simulink model "rfkjr"  (R2024a)
settings: Solver=FixedStepAuto  StartTime=0.0  StopTime=inf  FixedStep=0.1  RelTol=1e-3
libraries: robotlib x6
settings Model: Creator=ronnie.yalung  LastModifiedBy=ronnie.yalung
settings OptimizationCC: EnhancedBackFolding=on  PassReuseOutputArgsAs=Individual arguments  ZeroExternalMemoryAtStartup=off  ZeroInternalMemoryAtStartup=off  MaxStackSize=64  OptimizeBlockOrder=speed  DifferentSizesBufferReuse=on  OptimizationCustomize=off  EfficientTunableParamExpr=on
settings DebuggingCC: ParameterTunabilityLossMsg=error
settings HardwareCC: ProdBitPerLong=64  ProdHWDeviceType=Apple->ARM64  UseEmbeddedCoderFeatures=off
settings SFSimCC: MATLABDynamicMemAlloc=off
settings RTWCC: Description=Embedded Coder  SystemTargetFile=ert.tlc  HardwareBoard=Robot Operating System 2 (ROS 2)  TLCOptions="-aInlineSetEventsForThisBaseRateFcn=TLC_FALSE -aSuppressMultiTaskScheduler=TLC_FALSE  -aRateBasedStepFcn=0"  TemplateMakefile=ert_default_tmf  Toolchain=Colcon Tools  TargetLang=C++
settings CodeAppCC: ForceParamTrailComments=on  IgnoreCustomStorageClasses=off  OperatorAnnotations=on  SimulinkDataObjDesc=on  SFDataObjDesc=on  InsertBlockDesc=on
settings ERTTargetCC: CodeInterfacePackaging=C++ class  SupportNonInlinedSFcns=on

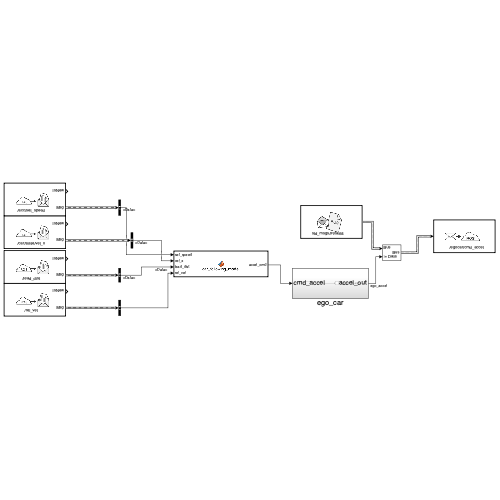
[thumbnail: Simulink's stored preview of the top-level diagram]
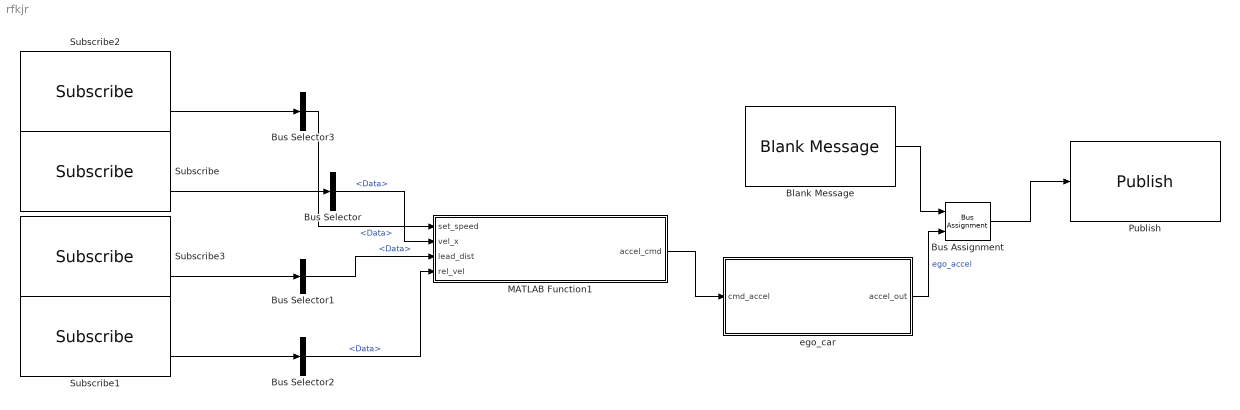
== system rfkjr ==
  Blank Message : robotlib/Blank Message  messageClass=Message  entityType=std_msgs/Float64  messageType=std_msgs/Float64  SampleTime=inf  legacyBusStruct=off
  Bus Assignment : BusAssignment  AssignedSignals=Data
  Bus Selector{,1..3} (4 alike) : BusSelector  OutputSignals=Data
  MATLAB Function1 : MATLAB Function  TreatAsAtomicUnit=on
  Publish : robotlib/Publish  topicSource=Specify your own  topic=/egocar/cmd_accel  messageType=std_msgs/Float64  legacyBusStruct=off  messageQueueLength=1
  Subscribe : robotlib/Subscribe  topicSource=Specify your own  topic=/car/state/vel_x  messageType=std_msgs/Float64  SampleTime=-1  legacyBusStruct=off  messageQueueLength=1
  Subscribe1 : robotlib/Subscribe  topicSource=Specify your own  topic=/rel_vel  messageType=std_msgs/Float64  SampleTime=-1  legacyBusStruct=off  messageQueueLength=1
  Subscribe2 : robotlib/Subscribe  topicSource=Specify your own  topic=/acc/set_speed  messageType=std_msgs/Int16  SampleTime=-1  legacyBusStruct=off  messageQueueLength=1
  Subscribe3 : robotlib/Subscribe  topicSource=Specify your own  topic=/lead_dist  messageType=std_msgs/Float64  SampleTime=-1  legacyBusStruct=off  messageQueueLength=1
  ego_car : Subsystem
  wires:
  MATLAB Function1/1(accel_cmd) -> ego_car/1(cmd_accel)
  Bus Assignment/1 -> Publish/1
  Blank Message/1 -> Bus Assignment/1
  ego_car/1(accel_out) -> Bus Assignment/2  "ego_accel"
  Subscribe/2 -> Bus Selector/1
  Bus Selector/1 -> MATLAB Function1/2(vel_x)  "<Data>"
  Subscribe3/2 -> Bus Selector1/1
  Bus Selector1/1 -> MATLAB Function1/3(lead_dist)  "<Data>"
  Subscribe1/2 -> Bus Selector2/1
  Bus Selector2/1 -> MATLAB Function1/4(rel_vel)  "<Data>"
  Subscribe2/2 -> Bus Selector3/1
  Bus Selector3/1 -> MATLAB Function1/1(set_speed)  "<Data>"

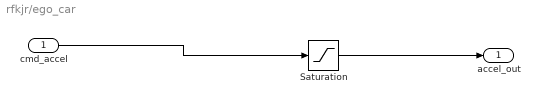
== system rfkjr/ego_car ==
  cmd_accel : Inport
  Saturation : Saturate  UpperLimit=5  LowerLimit=-5
  accel_out : Outport
  wires:
  Saturation/1 -> accel_out/1
  cmd_accel/1 -> Saturation/1

== matlab function rfkjr/MATLAB Function1 ==
  data: set_speed input; accel_cmd output; vel_x input; lead_dist input; rel_vel input
function accel_cmd = car_following_model(set_speed, vel_x, lead_dist, rel_vel)
    if set_speed == 0
        set_speed = int16(25);
    end
    
    % Parameters
    d_safe = 20; % Safe distance (meters)
    if set_speed > 50 %
        d_safe = 40;
    else 
        d_safe = 20;
    end
    
    kp = 2.0; % Proportional gain for distance
    kv = 1.0; % Proportional gain for relative velocity
    k_acc = 0.1; % Acceleration gain
    k_dec = 0.19; % Deceleration gain

    % Default value for accel_cmd
    accel_cmd = 0.0;  % Add a default assignment

    % Lead Car Proximity Logic
    if lead_dist < d_safe
        acc_lead = -kp * (d_safe - lead_dist) - kv * rel_vel;
        accel_cmd = acc_lead;  % Assign value for lead car condition
        return;
    end

    set_speed = double(set_speed); % convert to double for comparisons

    % Cruise Control Logic
    if vel_x < set_speed
        acc_cruise = k_acc * (set_speed - vel_x);
        accel_cmd = acc_cruise;  % Assign value for cruise control condition
    elseif vel_x > set_speed % Use double conversion only for the comparison
        acc_cruise = -k_dec * (vel_x - set_speed);
        accel_cmd = acc_cruise;  % Assign value for cruise control condition
    end
end
